simulink model "Simulink_model_171120bslee"  (R2017a)
settings: Solver=ode4  StartTime=0  StopTime=1500  FixedStep=0.01  RelTol=1e-3
model workspace (MAT data in the model file):
  A = 2
  Cd = 0.35
  Jm = 0.05
  Jt = 0.00226
  Jw = 0.905
  Ki = 0.083
  Kp = 0.24
  Nf = 4
  Ni = 2.3
  Rt = 0.316
  f = 0.01
  g = 9.81
  m = 1800
  rho = 1.166
  tout = [0; 1; 2; 3; 4; 5; 6; 7; 8; 9; 10; 11; 12; 13; 14; 15; 16; 17; 18; 19; 20; 21; 22; 23; 24; 25; 26; 27; 28; 29; 30; 31; 32; 33; 34; 35; 36; 37; 38; 39; 40; 41; 42; 43; 44; 45; 46; 47; 48; 49; 50]
  xxx = [0 1 2 3 4 5 6 7 8 9 10 11 ... (15447 elements, 1x15447)]
  yyy = [259 259 259 259 259 259 259 259 259 259 259 259 ... (15447 elements, 1x15447)]
libraries: simulink x1
(part 1 of 2)
settings Model: Creator=Peter lee  LastModifiedBy=dlqks
settings OptimizationCC: LifeSpan=inf
settings DebuggingCC: SFExecutionAtInitializationDiag=none

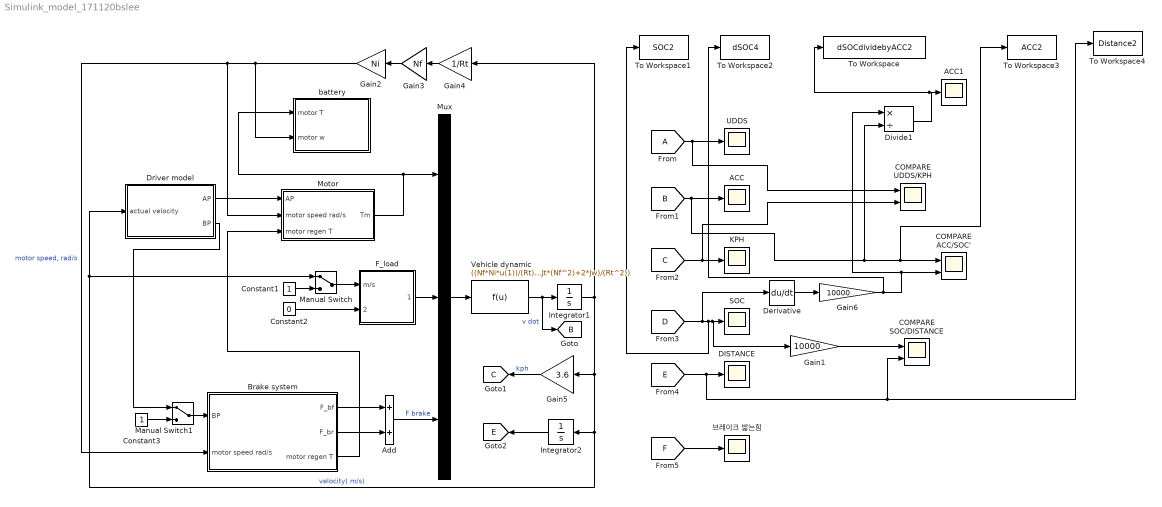
== system Simulink_model_171120bslee ==
  ACC : Scope
  ACC1 : Scope
  Add : Sum
  Brake system : Subsystem
  COMPARE ACC/SOC' : Scope  NumInputPorts=2
  COMPARE SOC/DISTANCE : Scope  NumInputPorts=2
  COMPARE UDDS/KPH : Scope  NumInputPorts=2
  Constant1 : Constant
  Constant2 : Constant  Value=0
  Constant3 : Constant
  DISTANCE : Scope
  Derivative : Derivative
  Divide1 : Product  Inputs=*/
  Driver model : Subsystem
  F_load : Subsystem
  Gain1 : Gain  Gain=10000
  Gain2 : Gain  Gain=Ni
  Gain3 : Gain  Gain=Nf
  Gain4 : Gain  Gain=1/Rt
  Gain5 : Gain  Gain=3.6
  Gain6 : Gain  Gain=10000
  Integrator1 : Integrator  InitialCondition=0.001
  Integrator2 : Integrator  InitialCondition=0.001
  KPH : Scope
  Manual Switch : ManualSwitch
  Manual Switch1 : ManualSwitch
  Motor : Subsystem
  Mux : Mux  Inputs=3
  SOC : Scope
  To Workspace : ToWorkspace  VariableName=dSOCdividebyACC2  SaveFormat=Timeseries  SampleTime=-1
  To Workspace1 : ToWorkspace  VariableName=SOC2  SaveFormat=Timeseries  SampleTime=-1
  To Workspace2 : ToWorkspace  VariableName=dSOC4  SaveFormat=Timeseries  SampleTime=-1
  To Workspace3 : ToWorkspace  VariableName=ACC2  SaveFormat=Timeseries  SampleTime=-1
  To Workspace4 : ToWorkspace  VariableName=Distance2  SaveFormat=Timeseries  SampleTime=-1
  UDDS : Scope
  Vehicle dynamic : Fcn  Expr=((Nf*Ni*u(1))/(Rt)-u(2)+u(3))/(m+(Jm*(Ni^2)*(Nf^2)+Jt*(Nf^2)+2*Jw)/(Rt^2))
  battery : Subsystem
  브레이크 밟는힘 : Scope
  tag scope: B=global, C=global, E=global
  wires:
  Integrator1/1 -> Gain5/1, Integrator2/1, Manual Switch/1, Driver model/1(actual velocity), Gain4/1  "velocity( m/s)"
  Mux/1 -> Vehicle dynamic/1
  Vehicle dynamic/1 -> [B], Integrator1/1  "v dot"
  Gain2/1 -> battery/2(motor w), Brake system/2(motor speed rad/s), Motor/2(motor speed rad/s)  "motor speed, rad/s"
  Gain4/1 -> Gain3/1
  Gain3/1 -> Gain2/1
  Gain5/1 -> [C]  "kph"
  Constant1/1 -> Manual Switch/2
  Constant3/1 -> Manual Switch1/2
  Add/1 -> Mux/3  "F brake"
  Manual Switch1/1 -> Brake system/1(BP)
  Brake system/1(F_bf) -> Add/1
  Brake system/2(F_br) -> Add/2
  Motor/1(Tm) -> battery/1(motor T), Mux/1
  Driver model/1("AP ") -> Motor/1(AP)
  Driver model/2(BP) -> Manual Switch1/1
  Manual Switch/1 -> F_load/1(m/s)
  F_load/1(F_load) -> Mux/2
  [D] -> To Workspace1/1, SOC/1, Gain1/1, Derivative/1
  Brake system/3(motor regen T) -> Motor/3(motor regen T)
  Constant2/1 -> F_load/2(Gradient)
  [A] -> UDDS/1, COMPARE UDDS/KPH/1
  [B] -> ACC/1, Divide1/2, COMPARE ACC/SOC'/1, To Workspace3/1
  [C] -> COMPARE UDDS/KPH/2, KPH/1
  Integrator2/1 -> [E]
  [E] -> COMPARE SOC/DISTANCE/2, To Workspace4/1, DISTANCE/1
  Gain1/1 -> COMPARE SOC/DISTANCE/1
  Gain6/1 -> To Workspace2/1, Divide1/1, COMPARE ACC/SOC'/2
  [F] -> 브레이크 밟는힘/1
  Divide1/1 -> To Workspace/1, ACC1/1
  Derivative/1 -> Gain6/1
